simulink model "Lab2"  (R2021b)
settings: Solver=VariableStepAuto  StartTime=0.0  StopTime=10.0  RelTol=1e-3
libraries: nesl_utility x14, fl_lib x12, ee_lib x7, eeRmsMeasurement x7
settings Model: Creator=coolk  LastModifiedBy=coolk

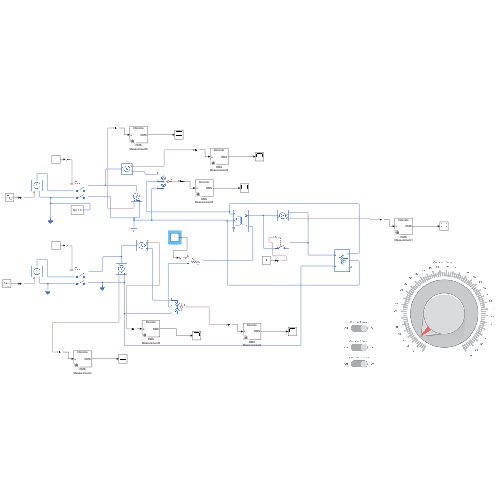
[thumbnail: Simulink's stored preview of the top-level diagram]
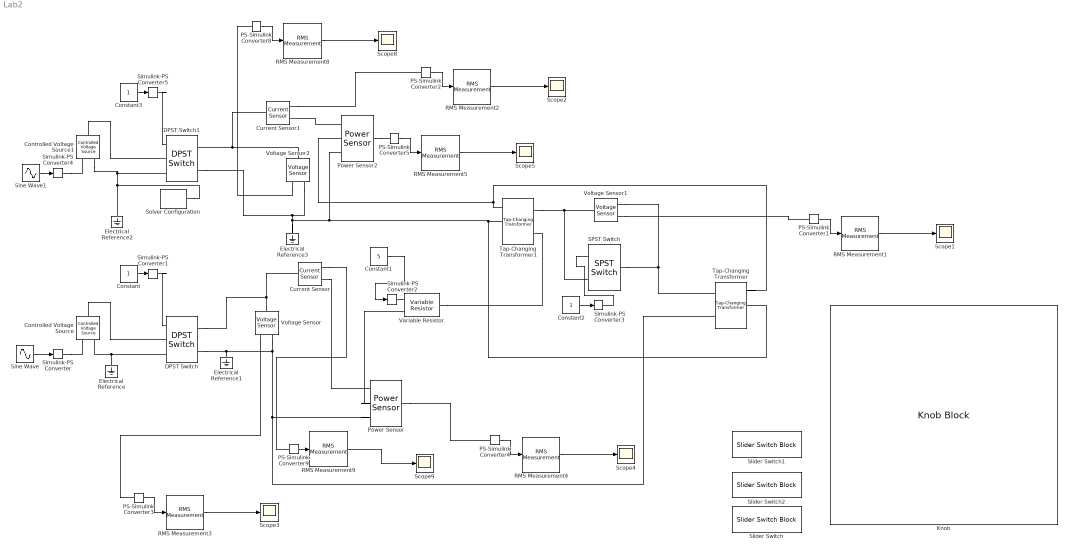
== system Lab2 ==
  Constant : Constant
  Constant1 : Constant  Value=5
  Constant2 : Constant
  Constant3 : Constant
  Controlled Voltage Source : fl_lib/Electrical/Electrical Sources/Controlled Voltage Source
  Controlled Voltage Source1 : fl_lib/Electrical/Electrical Sources/Controlled Voltage Source
  Current Sensor : fl_lib/Electrical/Electrical Sensors/Current Sensor
  Current Sensor1 : fl_lib/Electrical/Electrical Sensors/Current Sensor
  DPST Switch : ee_lib/Switches & Breakers/DPST Switch  R_closed=0.01 Ohm  G_open=1e-6 S  Threshold=0.5 V  Width=0 V  model_dynamics=0  t_on=1e-3 s  t_off=1e-3 s  initial_vT=0 V
      settings: SourceProductBaseCode=PS  InternalSimscapePortConfiguration="{\"Bottom\":[],\"Left\":[{\"id\":\"vT\",\"label\":\"vT\",\"type\":\"input\"},{\"id\":\"p1\",\"label\":\"\",\"type\":\"foundation.electrical.electrical\"},{\"id\":\"p2\",\"label\":\"\",\"type\":\"foundation.electrical.electrical\"}],\"Right\":[{\"id\":\"n1\",\"label\":\"\",\"type\":\"foundation.electrical.electrical\"},{\"id\":\"n2\",\"label\":\"\",\"type\":\"foundation.electrical.electrical\"}],\"Top\":[]}"
  DPST Switch1 : ee_lib/Switches & Breakers/DPST Switch  R_closed=0.01 Ohm  G_open=1e-6 S  Threshold=0.5 V  Width=0 V  model_dynamics=0  t_on=1e-3 s  t_off=1e-3 s  initial_vT=0 V
      settings: SourceProductBaseCode=PS  InternalSimscapePortConfiguration="{\"Bottom\":[],\"Left\":[{\"id\":\"vT\",\"label\":\"vT\",\"type\":\"input\"},{\"id\":\"p1\",\"label\":\"\",\"type\":\"foundation.electrical.electrical\"},{\"id\":\"p2\",\"label\":\"\",\"type\":\"foundation.electrical.electrical\"}],\"Right\":[{\"id\":\"n1\",\"label\":\"\",\"type\":\"foundation.electrical.electrical\"},{\"id\":\"n2\",\"label\":\"\",\"type\":\"foundation.electrical.electrical\"}],\"Top\":[]}"
  Electrical Reference{,1..3} (4 alike) : fl_lib/Electrical/Electrical Elements/Electrical Reference
  Knob : KnobBlock
  PS-Simulink Converter{1..5,8..9} (7 alike) : nesl_utility/PS-Simulink Converter  PhysicalDomain=network_engine_domain  SubClassName=ps_output  LeftPortType=input  RightPortType=output  PseudoPeriodic=off  Frequencies=[]  Unit=inherit  AffineConversion=off
      settings: SourceProductBaseCode=PW,SS
  Power Sensor : ee_lib/Sensors & Transducers/Power Sensor  measurement_type=1  averaging_period=1e-4 s
      settings: SourceProductBaseCode=PS
  Power Sensor2 : ee_lib/Sensors & Transducers/Power Sensor  measurement_type=1  averaging_period=1e-4 s
      settings: SourceProductBaseCode=PS
  RMS Measurement{1..5,8..9} (7 alike) : eeRmsMeasurement/RMS Measurement  LabelModeActiveChoice=Total  F=60  SpecifyHarmonics=off  K=[0 1 2]  Ts=10e-4
      settings: SourceProductBaseCode=PS
  SPST Switch : ee_lib/Switches & Breakers/SPST Switch  R_closed=0.01 Ohm  G_open=1e-6 S  Threshold=0.5 V  Width=0 V  model_dynamics=0  t_on=1e-3 s  t_off=1e-3 s  initial_vT=0 V
      settings: SourceProductBaseCode=PS  InternalSimscapePortConfiguration="{\"Bottom\":[],\"Left\":[{\"id\":\"vT\",\"label\":\"vT\",\"type\":\"input\"},{\"id\":\"p\",\"label\":\"\",\"type\":\"foundation.electrical.electrical\"}],\"Right\":[{\"id\":\"n\",\"label\":\"\",\"type\":\"foundation.electrical.electrical\"}],\"Top\":[]}"
  Scope{1..5,8..9} (7 alike) : Scope
  Simulink-PS Converter{,1..5} (6 alike) : nesl_utility/Simulink-PS Converter  PhysicalDomain=network_engine_domain  SubClassName=ps_input  LeftPortType=input  RightPortType=output  PseudoPeriodic=off  Frequencies=[]  NoiseDistribution=none  NoiseParameters=[]  Unit=1  AffineConversion=off  FilteringAndDerivatives=provide  SimscapeFilterOrder=1  InputFilterTimeConstant=0.001  UdotUserProvided=0
      settings: SourceProductBaseCode=PW,SS
  Sine Wave : Sin  Amplitude=28  SampleTime=0
  Sine Wave1 : Sin  Amplitude=325  SampleTime=0
  Slider Switch : SliderSwitchBlock
      settings: Values={{'Off', 'On'}, [0 1]}
  Slider Switch1 : SliderSwitchBlock
      settings: Values={{'Off', 'On'}, [0 1]}
  Slider Switch2 : SliderSwitchBlock
      settings: Values={{'Off', 'On'}, [0 1]}
  Solver Configuration : nesl_utility/Solver Configuration  PhysicalDomain=network_engine_domain  SubClassName=solver  LeftPortType=input  RightPortType=generic  Tones=[]  Harmonics=[]  SimulateNoise=off  Profile=off  UseLocalSampling=off  EnableSwitchedLinearOptims=on  FrequencyDomain=off  UseCCode=off  RelTol=0.001  AbsTol=1e-06  MinStep=1e-09  ToWorkspace=off  RevertToSquareIcSolve=off  NumHomotopyIterations=100  PhasorMode=off  PhasorModeNumHarmonics=1  DoDC=off  ResidualTolerance=1e-09  UseLocalSolver=off  LocalSolverChoice=NE_BACKWARD_EULER_ADVANCER  LocalSolverSampleTime=0.001  DoFixedCost=off  MaxNonlinIter=3  MaxModeIter=2  ComputeImpulses=off  ImpulseIterations=2  LinearAlgebra=auto  EquationFormulation=NE_TIME_EF  DelaysMemoryBudget=1024  AutomaticFiltering=on  FilteringTimeConstant=0.001  PartitionStorageMethod=AS_NEEDED  PartitionMemoryBudget=1024  PartitionMethod=ROBUST
      settings: SourceProductBaseCode=PW,SS
  Tap-Changing Transformer : ee_lib/Passive/Transformers/Tap-Changing Transformer  n0=1  Lp=1e-6 H  Ls=1e-6 H  Rm=1e6 Ohm  Lm=1 H  Rp=0 Ohm  Rs=1 Ohm  Gp=0 1/Ohm  Gs=0 1/Ohm  prm=1  pmin=-5  pmax=5  delta=1  controlThreshold=0.5  i1_specify=off  i1_priority=None  i1=0 A  i1_nominal_specify=off  i1_nominal_unit=A  i1_nominal_value=1  i2_specify=off  i2_priority=None  i2=0 A  i2_nominal_specify=off  i2_nominal_unit=A  i2_nominal_value=1  tapPosition_specify=off  tapPosition_priority=High  tapPosition=0
      settings: SourceProductBaseCode=PS  InternalSimscapePortConfiguration="{\"Bottom\":[],\"Left\":[{\"id\":\"p1\",\"label\":\"1+\",\"type\":\"foundation.electrical.electrical\"},{\"id\":\"n1\",\"label\":\"1-\",\"type\":\"foundation.electrical.electrical\"},{\"id\":\"control\",\"label\":\"c\",\"type\":\"input\"}],\"Right\":[{\"id\":\"p2\",\"label\":\"2+\",\"type\":\"foundation.electrical.electrical\"},{\"id\":\"n2\",\"label\":\"2-\",\"type\":\"foundation.electrical.electrical\"}],\"Top\":[]}"
  Tap-Changing Transformer1 : ee_lib/Passive/Transformers/Tap-Changing Transformer  n0=1  Lp=1e-6 H  Ls=1e-6 H  Rm=1e6 Ohm  Lm=1 H  Rp=0 Ohm  Rs=1 Ohm  Gp=0 1/Ohm  Gs=0 1/Ohm  prm=1  pmin=-5  pmax=5  delta=1  controlThreshold=0.5  i1_specify=off  i1_priority=None  i1=0 A  i1_nominal_specify=off  i1_nominal_unit=A  i1_nominal_value=1  i2_specify=off  i2_priority=None  i2=0 A  i2_nominal_specify=off  i2_nominal_unit=A  i2_nominal_value=1  tapPosition_specify=off  tapPosition_priority=High  tapPosition=0
      settings: SourceProductBaseCode=PS  InternalSimscapePortConfiguration="{\"Bottom\":[],\"Left\":[{\"id\":\"p1\",\"label\":\"1+\",\"type\":\"foundation.electrical.electrical\"},{\"id\":\"n1\",\"label\":\"1-\",\"type\":\"foundation.electrical.electrical\"},{\"id\":\"control\",\"label\":\"c\",\"type\":\"input\"}],\"Right\":[{\"id\":\"p2\",\"label\":\"2+\",\"type\":\"foundation.electrical.electrical\"},{\"id\":\"n2\",\"label\":\"2-\",\"type\":\"foundation.electrical.electrical\"}],\"Top\":[]}"
  Variable Resistor : fl_lib/Electrical/Electrical Elements/Variable Resistor  Rmin=0 Ohm  i_specify=off  i_priority=None  i=0 A  i_nominal_specify=off  i_nominal_unit=A  i_nominal_value=1  v_specify=off  v_priority=None  v=0 V  v_nominal_specify=off  v_nominal_unit=V  v_nominal_value=1
  Voltage Sensor : fl_lib/Electrical/Electrical Sensors/Voltage Sensor
  Voltage Sensor1 : fl_lib/Electrical/Electrical Sensors/Voltage Sensor
  Voltage Sensor2 : fl_lib/Electrical/Electrical Sensors/Voltage Sensor
  wires:
  Constant/1 -> Simulink-PS Converter1/1
  Constant1/1 -> Simulink-PS Converter2/1
  Constant2/1 -> Simulink-PS Converter3/1
  Sine Wave1/1 -> Simulink-PS Converter4/1
  Constant3/1 -> Simulink-PS Converter5/1
  RMS Measurement5/1 -> Scope5/1
  PS-Simulink Converter5/1 -> RMS Measurement5/1
  RMS Measurement1/1 -> Scope1/1
  PS-Simulink Converter1/1 -> RMS Measurement1/1
  RMS Measurement2/1 -> Scope2/1
  PS-Simulink Converter2/1 -> RMS Measurement2/1
  RMS Measurement3/1 -> Scope3/1
  PS-Simulink Converter3/1 -> RMS Measurement3/1
  RMS Measurement4/1 -> Scope4/1
  PS-Simulink Converter4/1 -> RMS Measurement4/1
  RMS Measurement8/1 -> Scope8/1
  PS-Simulink Converter8/1 -> RMS Measurement8/1
  RMS Measurement9/1 -> Scope9/1
  PS-Simulink Converter9/1 -> RMS Measurement9/1
  Sine Wave/1 -> Simulink-PS Converter/1
  connections:
  DPST Switch/LConn3 -- Electrical Reference/LConn1 -- Controlled Voltage Source/RConn2
  DPST Switch/RConn2 -- Voltage Sensor/RConn2 -- Power Sensor/LConn3 -- Tap-Changing Transformer/RConn2 -- Electrical Reference1/LConn1
  Simulink-PS Converter1/RConn1 -- DPST Switch/LConn1
  Controlled Voltage Source/LConn1 -- DPST Switch/LConn2
  DPST Switch/RConn1 -- Current Sensor/LConn1 -- Voltage Sensor/LConn1
  Current Sensor/RConn2 -- Power Sensor/LConn1
  Power Sensor/LConn2 -- Variable Resistor/LConn2
  Simulink-PS Converter2/RConn1 -- Variable Resistor/LConn1
  Variable Resistor/RConn1 -- Tap-Changing Transformer1/RConn2
  Tap-Changing Transformer1/RConn1 -- SPST Switch/LConn2 -- Voltage Sensor1/LConn1
  Voltage Sensor1/RConn2 -- Tap-Changing Transformer/RConn1 -- SPST Switch/RConn1
  SPST Switch/LConn1 -- Simulink-PS Converter3/RConn1
  Tap-Changing Transformer1/LConn2 -- DPST Switch1/RConn2 -- Voltage Sensor2/RConn2 -- Electrical Reference3/LConn1 -- Power Sensor2/LConn3 -- Tap-Changing Transformer/LConn2
  Tap-Changing Transformer/LConn1 -- Tap-Changing Transformer1/LConn1 -- Power Sensor2/LConn2
  Controlled Voltage Source1/RConn2 -- DPST Switch1/LConn3 -- Solver Configuration/RConn1 -- Electrical Reference2/LConn1
  Controlled Voltage Source1/LConn1 -- DPST Switch1/LConn2
  Simulink-PS Converter4/RConn1 -- Controlled Voltage Source1/RConn1
  Simulink-PS Converter5/RConn1 -- DPST Switch1/LConn1
  Current Sensor1/LConn1 -- DPST Switch1/RConn1 -- Voltage Sensor2/LConn1
  Power Sensor2/LConn1 -- Current Sensor1/RConn2
  Power Sensor2/RConn1 -- PS-Simulink Converter5/LConn1
  Voltage Sensor1/RConn1 -- PS-Simulink Converter1/LConn1
  Current Sensor1/RConn1 -- PS-Simulink Converter2/LConn1
  Voltage Sensor/RConn1 -- PS-Simulink Converter3/LConn1
  Power Sensor/RConn1 -- PS-Simulink Converter4/LConn1
  Voltage Sensor2/RConn1 -- PS-Simulink Converter8/LConn1
  Current Sensor/RConn1 -- PS-Simulink Converter9/LConn1
  Simulink-PS Converter/RConn1 -- Controlled Voltage Source/RConn1
